simulink model "Copy_of_cantoni_combined_matrices_3pools_gates_hil"  (R2019b)
settings: Solver=FixedStepDiscrete  StartTime=0.0  StopTime=60*30  FixedStep=1/SPS  RelTol=1e-3
undefined symbols (not defined in the file or in its folder): ddelay, LF, Pd, Pd0, serial, SPS, Wis
libraries: instrumentlib x12, hdlsllib x4, simulink x4, sldrtlib x1
settings Model: Creator=Jacob  LastModifiedBy=bas
settings DataIOCC: ReturnWorkspaceOutputs=off
settings SFSimCC: CustomCodeUndefinedFunction=UseInterfaceOnly

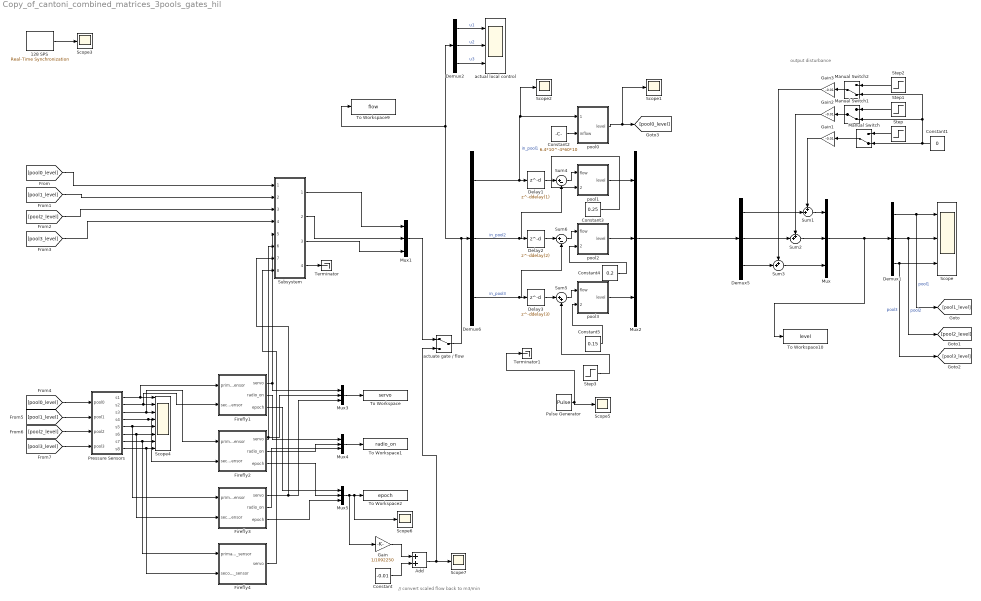
== system Copy_of_cantoni_combined_matrices_3pools_gates_hil ==
  note: // convert scaled flow back to m3/min
  note: output disturbance
  128 SPS : sldrtlib/Real-Time Synchronization  SampleTime=1/SPS  MaxMissedTicks=inf  ShowMissedTicks=on  YieldWhenWaiting=off
  Add : Sum
  Constant : Constant  Value=-0.01
  Constant1 : Constant  Value=0
  Constant2 : Constant  Value=6.4*10^-4*60*10
  Constant3 : Constant  Value=0.25  SampleTime=-1
  Constant4 : Constant  Value=0.2
  Constant5 : Constant  Value=0.15
  Delay1 : Delay  DelayLength=ddelay(1)
  Delay2 : Delay  DelayLength=ddelay(2)
  Delay3 : Delay  DelayLength=ddelay(3)
  Demux{1..2,5..6} (4 alike) : Demux  Outputs=3
  Firefly1 : Subsystem
  Firefly2 : Subsystem
  Firefly3 : Subsystem
  Firefly4 : Subsystem
  Gain : Gain  Gain=1/1092250
  Gain1 : Gain  Gain=-0.01
  Gain2 : Gain  Gain=-0.01
  Gain3 : Gain  Gain=-0.01
  Manual Switch : ManualSwitch  CurrentSetting=0
  Manual Switch1 : ManualSwitch  CurrentSetting=0
  Manual Switch2 : ManualSwitch  CurrentSetting=0
  Mux{,1..5} (6 alike) : Mux  Inputs=3
  Pressure Sensors : Subsystem
  Pulse Generator : DiscretePulseGenerator  Amplitude=-0.015  Period=60  PulseWidth=10
  Scope : Scope  NumInputPorts=3
  Scope{1..3,5..7} (6 alike) : Scope
  Scope4 : Scope  NumInputPorts=8
  Step : Step  Time=50  SampleTime=0
  Step1 : Step  Time=50  SampleTime=0
  Step2 : Step  Time=50  SampleTime=0
  Step3 : Step  Time=20  After=-0.015  SampleTime=0
  Subsystem : Subsystem
  Sum1 : Sum  Inputs=++|
  Sum2 : Sum  Inputs=++|
  Sum3 : Sum  Inputs=++|
  Sum4 : Sum  Inputs=|+-
  Sum5 : Sum  Inputs=|++
  Sum6 : Sum  Inputs=|+-
  Terminator : Terminator
  Terminator1 : Terminator
  To Workspace : ToWorkspace  VariableName=servo  SaveFormat=Timeseries  SampleTime=-1
  To Workspace1 : ToWorkspace  VariableName=radio_on  SaveFormat=Timeseries  SampleTime=-1
  To Workspace10 : ToWorkspace  VariableName=level  SaveFormat=Timeseries  SampleTime=-1
  To Workspace2 : ToWorkspace  VariableName=epoch  SaveFormat=Timeseries  SampleTime=-1
  To Workspace9 : ToWorkspace  VariableName=flow  SaveFormat=Timeseries  SampleTime=-1
  actual local control : Scope  NumInputPorts=3
  actuate gate / flow : ManualSwitch
  pool0 : Subsystem
  pool1 : Subsystem
  pool2 : Subsystem
  pool3 : Subsystem
  wires:
  Demux1/1 -> Scope/1, [pool1_level]  "pool1"
  Demux1/2 -> [pool2_level], Scope/2  "pool2"
  Demux1/3 -> [pool3_level], Scope/3  "pool3"
  Step/1 -> Manual Switch/1
  Sum1/1 -> Mux/1
  Sum2/1 -> Mux/2
  Gain2/1 -> Sum2/1
  Step1/1 -> Manual Switch1/1
  Gain1/1 -> Sum1/1
  Manual Switch/1 -> Gain1/1
  Constant1/1 -> Manual Switch1/2, Manual Switch2/2, Manual Switch/2
  Manual Switch1/1 -> Gain2/1
  Sum3/1 -> Mux/3
  Manual Switch2/1 -> Gain3/1
  Step2/1 -> Manual Switch2/1
  Gain3/1 -> Sum3/1
  Demux5/1 -> Sum1/2
  Demux5/2 -> Sum2/2
  Demux5/3 -> Sum3/2
  Delay1/1 -> Sum4/1
  Delay2/1 -> Sum6/1
  Demux6/1 -> Scope2/1, pool0/1(outflow), Delay1/1  "in_pool1"
  Demux6/2 -> Sum4/2, Delay2/1  "in_pool2"
  Demux6/3 -> Sum6/2, Delay3/1  "in_pool3"
  Sum4/1 -> pool1/1(flow)
  pool1/1(level) -> Mux2/1
  Sum6/1 -> pool2/1(flow)
  pool2/1(level) -> Mux2/2
  Delay3/1 -> Sum5/1
  pool3/1(level) -> Mux2/3
  Demux2/3 -> actual local control/3  "u3"
  Demux2/1 -> actual local control/1  "u1"
  Demux2/2 -> actual local control/2  "u2"
  actuate gate / flow/1 -> To Workspace9/1, Demux2/1, Demux6/1
  pool0/1(level) -> Scope1/1, [pool0_level]
  [pool0_level] -> Subsystem/1(pool0)
  [pool1_level] -> Subsystem/2(pool1)
  [pool2_level] -> Subsystem/3(pool2)
  [pool3_level] -> Subsystem/4(pool3)
  Constant2/1 -> pool0/2(inflow)
  Sum5/1 -> pool3/1(flow)
  Pulse Generator/1 -> Terminator1/1, Scope5/1
  Mux/1 -> To Workspace10/1, Demux1/1
  Pressure Sensors/1(s1) -> Firefly1/1(primary_sensor), Scope4/1
  Pressure Sensors/2(s2) -> Firefly1/2(secondary_sensor), Scope4/2
  Pressure Sensors/3(s3) -> Firefly2/1(primary_sensor), Scope4/3
  Pressure Sensors/4(s4) -> Firefly2/2(secondary_sensor), Scope4/4
  Pressure Sensors/5(s5) -> Firefly3/1(primary_sensor), Scope4/5
  Pressure Sensors/6(s6) -> Firefly3/2(secondary_sensor), Scope4/6
  Pressure Sensors/7(s7) -> Firefly4/1(primary_sensor), Scope4/7
  Pressure Sensors/8(s8) -> Firefly4/2(secondary_sensor), Scope4/8
  [pool0_level] -> Pressure Sensors/1(pool0)
  [pool1_level] -> Pressure Sensors/2(pool1)
  [pool2_level] -> Pressure Sensors/3(pool2)
  [pool3_level] -> Pressure Sensors/4(pool3)
  Subsystem/1(flow0_1) -> Mux1/1
  Subsystem/2(flow1_2) -> Mux1/2
  Subsystem/3(flow2_3) -> Mux1/3
  Subsystem/4(flow3_4) -> Terminator/1
  Mux2/1 -> Demux5/1
  Firefly1/1("servo ") -> Subsystem/5(servo1), Mux3/1
  Firefly4/1("servo ") -> Subsystem/8(servo4)
  128 SPS/1 -> Scope3/1
  Constant5/1 -> pool3/2("initail_level ")
  Constant4/1 -> pool2/2(initial_level)
  Constant3/1 -> pool1/2(initial_level)
  Firefly3/1("servo ") -> Mux3/3, Subsystem/7(servo3)
  Mux3/1 -> To Workspace/1
  Mux4/1 -> To Workspace1/1
  Mux5/1 -> Gain/1, Scope6/1, To Workspace2/1
  Firefly1/2(radio_on) -> Mux4/1
  Firefly1/3(epoch) -> Mux5/1
  Firefly2/1("servo ") -> Mux3/2, Subsystem/6(servo2)
  Firefly2/2(radio_on) -> Mux4/2
  Firefly2/3(epoch) -> Mux5/2
  Firefly3/2(radio_on) -> Mux4/3
  Firefly3/3(epoch) -> Mux5/3
  Step3/1 -> Sum5/2
  Gain/1 -> Add/1
  Constant/1 -> Add/2
  Add/1 -> actuate gate / flow/2, Scope7/1
  Mux1/1 -> actuate gate / flow/1

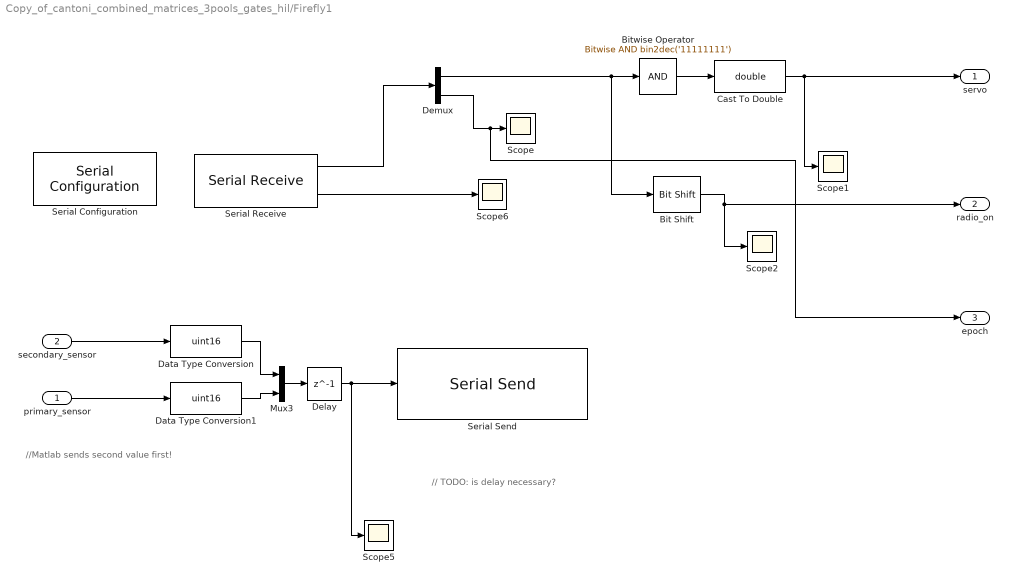
== system Copy_of_cantoni_combined_matrices_3pools_gates_hil/Firefly1 ==
  note: // TODO: is delay necessary?
  note: //Matlab sends second value first!
  primary_sensor : Inport
  secondary_sensor : Inport  Port=2
  Bit Shift : hdlsllib/Logic and Bit Operations/Bit Shift  mode=Shift Right Logical  N=8
      settings: SourceProductName=Simulink
  Bitwise Operator : simulink/Logic and Bit Operations/Bitwise Operator  logicop=AND  UseBitMask=on  BitMask=bin2dec('11111111')  BitMaskRealWorld=Stored Integer
  Cast To Double : DataTypeConversion  OutDataTypeStr=double
  Data Type Conversion : DataTypeConversion  OutDataTypeStr=uint16
  Data Type Conversion1 : DataTypeConversion  OutDataTypeStr=uint16
  Delay : Delay  DelayLength=1
  Demux : Demux  Outputs=2
  Mux3 : Mux  Inputs=2
  Scope{,1..2,5..6} (5 alike) : Scope
  Serial Configuration : instrumentlib/Serial Configuration  Priority=-200000  ComPortMenu=<Please select a port...>  ComPort=/dev/cu.SLAB_USBtoUART  ObjConstructor=serial('/dev/cu.SLAB_USBtoUART');  BaudRate=460800  DataBits=8  Parity=none  StopBits=1  FlowControl=none  Timeout=10  ByteOrder=BigEndian
  Serial Receive : instrumentlib/Serial Receive  ComPortMenu=<Please select a port...>  ComPort=/dev/cu.SLAB_USBtoUART  ObjConstructor=serial('/dev/cu.SLAB_USBtoUART');  Terminator=<none>  DataSize="[2  1]"  DataType=uint16  EnableBlockingMode=off  ActionDataUnavailable=Output last received value  CustomValue=0  SampleTime=1/SPS
  Serial Send : instrumentlib/Serial Send  ComPortMenu=<Please select a port...>  ComPort=/dev/cu.SLAB_USBtoUART  ObjConstructor=serial('/dev/cu.SLAB_USBtoUART');  Header=#  Terminator=LF ('\n')  EnableBlockingMode=off
  "servo " : Outport
  radio_on : Outport  Port=2
  epoch : Outport  Port=3
  wires:
  Data Type Conversion1/1 -> Mux3/2
  primary_sensor/1 -> Data Type Conversion1/1
  secondary_sensor/1 -> Data Type Conversion/1
  Serial Receive/2 -> Scope6/1
  Mux3/1 -> Delay/1
  Delay/1 -> Serial Send/1, Scope5/1
  Data Type Conversion/1 -> Mux3/1
  Demux/2 -> epoch/1, Scope/1
  Serial Receive/1 -> Demux/1
  Cast To Double/1 -> Scope1/1, "servo "/1
  Demux/1 -> Bit Shift/1, Bitwise Operator/1
  Bitwise Operator/1 -> Cast To Double/1
  Bit Shift/1 -> radio_on/1, Scope2/1

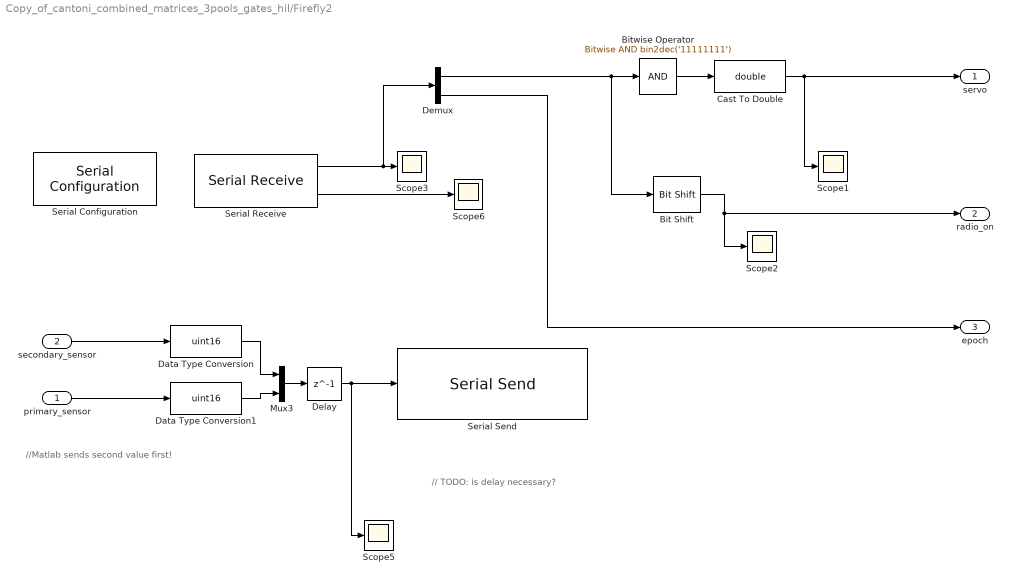
== system Copy_of_cantoni_combined_matrices_3pools_gates_hil/Firefly2 ==
  note: // TODO: is delay necessary?
  note: //Matlab sends second value first!
  primary_sensor : Inport
  secondary_sensor : Inport  Port=2
  Bit Shift : hdlsllib/Logic and Bit Operations/Bit Shift  mode=Shift Right Logical  N=8
      settings: SourceProductName=Simulink
  Bitwise Operator : simulink/Logic and Bit Operations/Bitwise Operator  logicop=AND  UseBitMask=on  BitMask=bin2dec('11111111')  BitMaskRealWorld=Stored Integer
  Cast To Double : DataTypeConversion  OutDataTypeStr=double
  Data Type Conversion : DataTypeConversion  OutDataTypeStr=uint16
  Data Type Conversion1 : DataTypeConversion  OutDataTypeStr=uint16
  Delay : Delay  DelayLength=1
  Demux : Demux  Outputs=2
  Mux3 : Mux  Inputs=2
  Scope{1..3,5..6} (5 alike) : Scope
  Serial Configuration : instrumentlib/Serial Configuration  Priority=-200000  ComPortMenu=<Please select a port...>  ComPort=/dev/cu.SLAB_USBtoUART4  ObjConstructor=serial('/dev/cu.SLAB_USBtoUART4');  BaudRate=460800  DataBits=8  Parity=none  StopBits=1  FlowControl=none  Timeout=10  ByteOrder=BigEndian
  Serial Receive : instrumentlib/Serial Receive  ComPortMenu=<Please select a port...>  ComPort=/dev/cu.SLAB_USBtoUART4  ObjConstructor=serial('/dev/cu.SLAB_USBtoUART4');  Terminator=<none>  DataSize="[2  1]"  DataType=uint16  EnableBlockingMode=off  ActionDataUnavailable=Output last received value  CustomValue=0  SampleTime=1/SPS
  Serial Send : instrumentlib/Serial Send  ComPortMenu=<Please select a port...>  ComPort=/dev/cu.SLAB_USBtoUART4  ObjConstructor=serial('/dev/cu.SLAB_USBtoUART4');  Header=#  Terminator=LF ('\n')  EnableBlockingMode=off
  "servo " : Outport
  radio_on : Outport  Port=2
  epoch : Outport  Port=3
  wires:
  Data Type Conversion1/1 -> Mux3/2
  primary_sensor/1 -> Data Type Conversion1/1
  secondary_sensor/1 -> Data Type Conversion/1
  Serial Receive/2 -> Scope6/1
  Mux3/1 -> Delay/1
  Delay/1 -> Serial Send/1, Scope5/1
  Data Type Conversion/1 -> Mux3/1
  Serial Receive/1 -> Demux/1, Scope3/1
  Cast To Double/1 -> Scope1/1, "servo "/1
  Demux/1 -> Bit Shift/1, Bitwise Operator/1
  Bitwise Operator/1 -> Cast To Double/1
  Demux/2 -> epoch/1
  Bit Shift/1 -> radio_on/1, Scope2/1

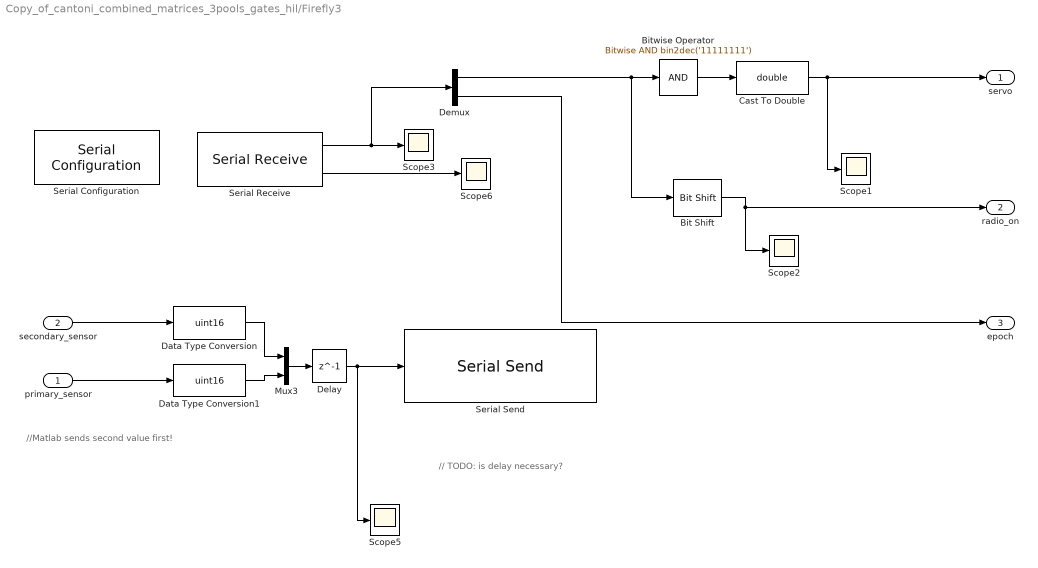
== system Copy_of_cantoni_combined_matrices_3pools_gates_hil/Firefly3 ==
  note: // TODO: is delay necessary?
  note: //Matlab sends second value first!
  primary_sensor : Inport
  secondary_sensor : Inport  Port=2
  Bit Shift : hdlsllib/Logic and Bit Operations/Bit Shift  mode=Shift Right Logical  N=8
      settings: SourceProductName=Simulink
  Bitwise Operator : simulink/Logic and Bit Operations/Bitwise Operator  logicop=AND  UseBitMask=on  BitMask=bin2dec('11111111')  BitMaskRealWorld=Stored Integer
  Cast To Double : DataTypeConversion  OutDataTypeStr=double
  Data Type Conversion : DataTypeConversion  OutDataTypeStr=uint16
  Data Type Conversion1 : DataTypeConversion  OutDataTypeStr=uint16
  Delay : Delay  DelayLength=1
  Demux : Demux  Outputs=2
  Mux3 : Mux  Inputs=2
  Scope{1..3,5..6} (5 alike) : Scope
  Serial Configuration : instrumentlib/Serial Configuration  Priority=-200000  ComPortMenu=<Please select a port...>  ComPort=/dev/cu.SLAB_USBtoUART6  ObjConstructor=serial('/dev/cu.SLAB_USBtoUART6');  BaudRate=460800  DataBits=8  Parity=none  StopBits=1  FlowControl=none  Timeout=10  ByteOrder=BigEndian
  Serial Receive : instrumentlib/Serial Receive  ComPortMenu=<Please select a port...>  ComPort=/dev/cu.SLAB_USBtoUART6  ObjConstructor=serial('/dev/cu.SLAB_USBtoUART6');  Terminator=<none>  DataSize="[2  1]"  DataType=uint16  EnableBlockingMode=off  ActionDataUnavailable=Output last received value  CustomValue=0  SampleTime=1/SPS
  Serial Send : instrumentlib/Serial Send  ComPortMenu=<Please select a port...>  ComPort=/dev/cu.SLAB_USBtoUART6  ObjConstructor=serial('/dev/cu.SLAB_USBtoUART6');  Header=#  Terminator=LF ('\n')  EnableBlockingMode=off
  "servo " : Outport
  radio_on : Outport  Port=2
  epoch : Outport  Port=3
  wires:
  Serial Receive/1 -> Demux/1, Scope3/1
  Data Type Conversion1/1 -> Mux3/2
  primary_sensor/1 -> Data Type Conversion1/1
  secondary_sensor/1 -> Data Type Conversion/1
  Serial Receive/2 -> Scope6/1
  Mux3/1 -> Delay/1
  Delay/1 -> Serial Send/1, Scope5/1
  Data Type Conversion/1 -> Mux3/1
  Cast To Double/1 -> Scope1/1, "servo "/1
  Demux/1 -> Bit Shift/1, Bitwise Operator/1
  Bitwise Operator/1 -> Cast To Double/1
  Demux/2 -> epoch/1
  Bit Shift/1 -> radio_on/1, Scope2/1

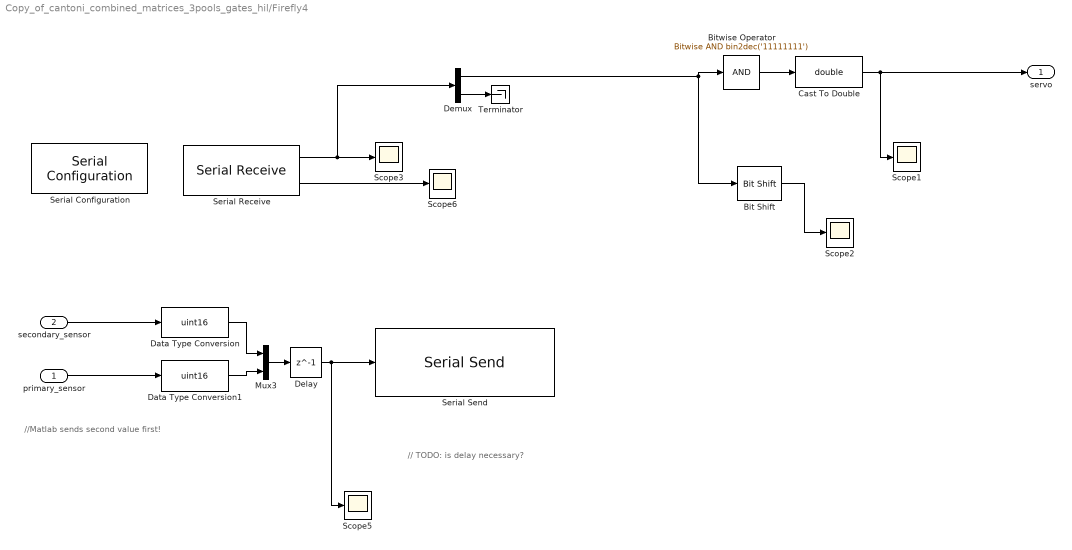
== system Copy_of_cantoni_combined_matrices_3pools_gates_hil/Firefly4 ==
  note: // TODO: is delay necessary?
  note: //Matlab sends second value first!
  primary_sensor : Inport
  secondary_sensor : Inport  Port=2
  Bit Shift : hdlsllib/Logic and Bit Operations/Bit Shift  mode=Shift Right Logical  N=8
      settings: SourceProductName=Simulink
  Bitwise Operator : simulink/Logic and Bit Operations/Bitwise Operator  logicop=AND  UseBitMask=on  BitMask=bin2dec('11111111')  BitMaskRealWorld=Stored Integer
  Cast To Double : DataTypeConversion  OutDataTypeStr=double
  Data Type Conversion : DataTypeConversion  OutDataTypeStr=uint16
  Data Type Conversion1 : DataTypeConversion  OutDataTypeStr=uint16
  Delay : Delay  DelayLength=1
  Demux : Demux  Outputs=2
  Mux3 : Mux  Inputs=2
  Scope{1..3,5..6} (5 alike) : Scope
  Serial Configuration : instrumentlib/Serial Configuration  Priority=-200000  ComPortMenu=<Please select a port...>  ComPort=/dev/cu.SLAB_USBtoUART8  ObjConstructor=serial('/dev/cu.SLAB_USBtoUART8');  BaudRate=460800  DataBits=8  Parity=none  StopBits=1  FlowControl=none  Timeout=10  ByteOrder=BigEndian
  Serial Receive : instrumentlib/Serial Receive  ComPortMenu=<Please select a port...>  ComPort=/dev/cu.SLAB_USBtoUART8  ObjConstructor=serial('/dev/cu.SLAB_USBtoUART8');  Terminator=<none>  DataSize="[2  1]"  DataType=uint16  EnableBlockingMode=off  ActionDataUnavailable=Output last received value  CustomValue=0  SampleTime=1/SPS
  Serial Send : instrumentlib/Serial Send  ComPortMenu=<Please select a port...>  ComPort=/dev/cu.SLAB_USBtoUART8  ObjConstructor=serial('/dev/cu.SLAB_USBtoUART8');  Header=#  Terminator=LF ('\n')  EnableBlockingMode=off
  Terminator : Terminator
  "servo " : Outport
  wires:
  Serial Receive/1 -> Demux/1, Scope3/1
  Data Type Conversion1/1 -> Mux3/2
  primary_sensor/1 -> Data Type Conversion1/1
  secondary_sensor/1 -> Data Type Conversion/1
  Serial Receive/2 -> Scope6/1
  Mux3/1 -> Delay/1
  Delay/1 -> Serial Send/1, Scope5/1
  Data Type Conversion/1 -> Mux3/1
  Demux/2 -> Terminator/1
  Cast To Double/1 -> Scope1/1, "servo "/1
  Demux/1 -> Bitwise Operator/1, Bit Shift/1
  Bit Shift/1 -> Scope2/1
  Bitwise Operator/1 -> Cast To Double/1

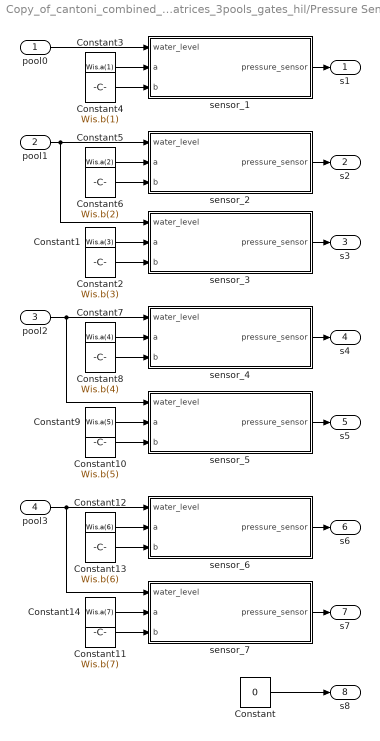
== system Copy_of_cantoni_combined_matrices_3pools_gates_hil/Pressure Sensors ==
  pool0 : Inport
  pool1 : Inport  Port=2
  pool2 : Inport  Port=3
  pool3 : Inport  Port=4
  Constant : Constant  Value=0
  Constant1 : Constant  Value=Wis.a(3)
  Constant10 : Constant  Value=Wis.b(5)
  Constant11 : Constant  Value=Wis.b(7)
  Constant12 : Constant  Value=Wis.a(6)
  Constant13 : Constant  Value=Wis.b(6)
  Constant14 : Constant  Value=Wis.a(7)
  Constant2 : Constant  Value=Wis.b(3)
  Constant3 : Constant  Value=Wis.a(1)
  Constant4 : Constant  Value=Wis.b(1)
  Constant5 : Constant  Value=Wis.a(2)
  Constant6 : Constant  Value=Wis.b(2)
  Constant7 : Constant  Value=Wis.a(4)
  Constant8 : Constant  Value=Wis.b(4)
  Constant9 : Constant  Value=Wis.a(5)
  sensor_1 : MATLAB Function  TreatAsAtomicUnit=on
  sensor_2 : MATLAB Function  TreatAsAtomicUnit=on
  sensor_3 : MATLAB Function  TreatAsAtomicUnit=on
  sensor_4 : MATLAB Function  TreatAsAtomicUnit=on
  sensor_5 : MATLAB Function  TreatAsAtomicUnit=on
  sensor_6 : MATLAB Function  TreatAsAtomicUnit=on
  sensor_7 : MATLAB Function  TreatAsAtomicUnit=on
  s1 : Outport
  s2 : Outport  Port=2
  s3 : Outport  Port=3
  s4 : Outport  Port=4
  s5 : Outport  Port=5
  s6 : Outport  Port=6
  s7 : Outport  Port=7
  s8 : Outport  Port=8
  wires:
  sensor_1/1(pressure_sensor) -> s1/1
  Constant5/1 -> sensor_2/2(a)
  Constant3/1 -> sensor_1/2(a)
  Constant4/1 -> sensor_1/3(b)
  Constant6/1 -> sensor_2/3(b)
  sensor_2/1(pressure_sensor) -> s2/1
  pool0/1 -> sensor_1/1(water_level)
  Constant1/1 -> sensor_3/2(a)
  Constant2/1 -> sensor_3/3(b)
  sensor_3/1(pressure_sensor) -> s3/1
  sensor_4/1(pressure_sensor) -> s4/1
  Constant7/1 -> sensor_4/2(a)
  Constant8/1 -> sensor_4/3(b)
  Constant10/1 -> sensor_5/3(b)
  Constant9/1 -> sensor_5/2(a)
  pool2/1 -> sensor_5/1(water_level), sensor_4/1(water_level)
  sensor_5/1(pressure_sensor) -> s5/1
  Constant12/1 -> sensor_6/2(a)
  pool3/1 -> sensor_7/1(water_level), sensor_6/1(water_level)
  sensor_6/1(pressure_sensor) -> s6/1
  Constant13/1 -> sensor_6/3(b)
  Constant11/1 -> sensor_7/3(b)
  Constant14/1 -> sensor_7/2(a)
  sensor_7/1(pressure_sensor) -> s7/1
  Constant/1 -> s8/1
  pool1/1 -> sensor_3/1(water_level), sensor_2/1(water_level)

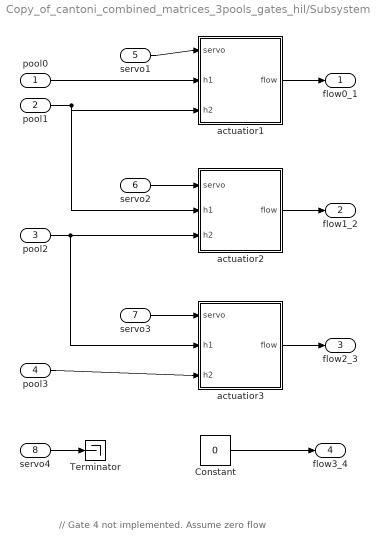
== system Copy_of_cantoni_combined_matrices_3pools_gates_hil/Subsystem ==
  note: // Gate 4 not implemented. Assume zero flow
  pool0 : Inport
  pool1 : Inport  Port=2
  pool2 : Inport  Port=3
  pool3 : Inport  Port=4
  servo1 : Inport  Port=5
  servo2 : Inport  Port=6
  servo3 : Inport  Port=7
  servo4 : Inport  Port=8
  Constant : Constant  Value=0
  Terminator : Terminator
  actuatior1 : MATLAB Function  TreatAsAtomicUnit=on
  actuatior2 : MATLAB Function  TreatAsAtomicUnit=on
  actuatior3 : MATLAB Function  TreatAsAtomicUnit=on
  flow0_1 : Outport
  flow1_2 : Outport  Port=2
  flow2_3 : Outport  Port=3
  flow3_4 : Outport  Port=4
  wires:
  pool1/1 -> actuatior2/2(h1), actuatior1/3(h2)
  servo2/1 -> actuatior2/1(servo)
  pool2/1 -> actuatior3/2(h1), actuatior2/3(h2)
  actuatior1/1(flow) -> flow0_1/1
  servo1/1 -> actuatior1/1(servo)
  servo3/1 -> actuatior3/1(servo)
  pool0/1 -> actuatior1/2(h1)
  actuatior2/1(flow) -> flow1_2/1
  pool3/1 -> actuatior3/3(h2)
  actuatior3/1(flow) -> flow2_3/1
  servo4/1 -> Terminator/1
  Constant/1 -> flow3_4/1

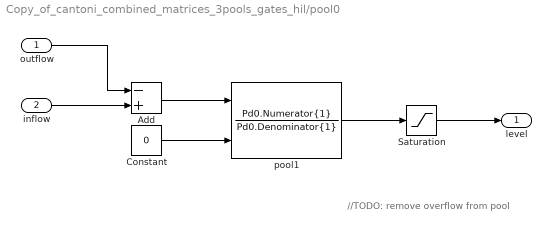
== system Copy_of_cantoni_combined_matrices_3pools_gates_hil/pool0 ==
  note: //TODO: remove overflow from pool
  outflow : Inport
  inflow : Inport  Port=2
  Add : Sum  Inputs=-+
  Constant : Constant  Value=0
  Saturation : Saturate  UpperLimit=0.3
  pool1 : DiscreteTransferFcn  Numerator=Pd0.Numerator{1}  Denominator=Pd0.Denominator{1}  InitialStatesSource=Input port
      settings: InputPortMap=u0,p5
  level : Outport
  wires:
  pool1/1 -> Saturation/1
  outflow/1 -> Add/1
  inflow/1 -> Add/2
  Add/1 -> pool1/1
  Constant/1 -> pool1/2
  Saturation/1 -> level/1

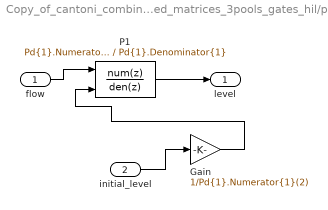
== system Copy_of_cantoni_combined_matrices_3pools_gates_hil/pool1 ==
  flow : Inport
  initial_level : Inport  Port=2
  Gain : Gain  Gain=1/Pd{1}.Numerator{1}(2)
  P1 : DiscreteTransferFcn  Numerator=Pd{1}.Numerator{1}  Denominator=Pd{1}.Denominator{1}  InitialStatesSource=Input port
      settings: InputPortMap=u0,p5
  level : Outport
  wires:
  flow/1 -> P1/1
  P1/1 -> level/1
  Gain/1 -> P1/2
  initial_level/1 -> Gain/1

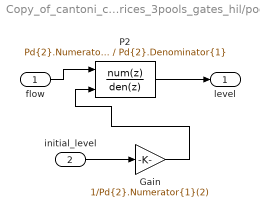
== system Copy_of_cantoni_combined_matrices_3pools_gates_hil/pool2 ==
  flow : Inport
  initial_level : Inport  Port=2
  Gain : Gain  Gain=1/Pd{2}.Numerator{1}(2)
  P2 : DiscreteTransferFcn  Numerator=Pd{2}.Numerator{1}  Denominator=Pd{2}.Denominator{1}  InitialStatesSource=Input port
      settings: InputPortMap=u0,p5
  level : Outport
  wires:
  flow/1 -> P2/1
  P2/1 -> level/1
  Gain/1 -> P2/2
  initial_level/1 -> Gain/1

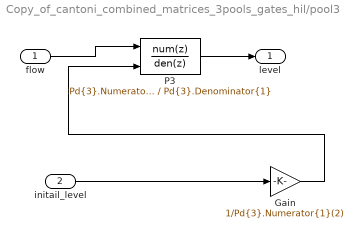
== system Copy_of_cantoni_combined_matrices_3pools_gates_hil/pool3 ==
  flow : Inport
  "initail_level " : Inport  Port=2
  Gain : Gain  Gain=1/Pd{3}.Numerator{1}(2)
  P3 : DiscreteTransferFcn  Numerator=Pd{3}.Numerator{1}  Denominator=Pd{3}.Denominator{1}  InitialStatesSource=Input port
      settings: InputPortMap=u0,p5
  level : Outport
  wires:
  P3/1 -> level/1
  flow/1 -> P3/1
  Gain/1 -> P3/2
  "initail_level "/1 -> Gain/1

== matlab function Copy_of_cantoni_combined_matrices_3pools_gates_hil/Pressure Sensors/sensor_1 ==
  data: water_level input; pressure_sensor output; a input; b input
function pressure_sensor = fcn(water_level, a, b)

pressure_sensor = m2pressure(water_level, a, b);

== matlab function Copy_of_cantoni_combined_matrices_3pools_gates_hil/Pressure Sensors/sensor_2 ==
  data: water_level input; pressure_sensor output; a input; b input
function pressure_sensor = fcn(water_level, a, b)

pressure_sensor = m2pressure(water_level, a, b);

== matlab function Copy_of_cantoni_combined_matrices_3pools_gates_hil/Pressure Sensors/sensor_3 ==
  data: water_level input; pressure_sensor output; a input; b input
function pressure_sensor = fcn(water_level, a, b)

pressure_sensor = m2pressure(water_level, a, b);

== matlab function Copy_of_cantoni_combined_matrices_3pools_gates_hil/Pressure Sensors/sensor_4 ==
  data: water_level input; pressure_sensor output; a input; b input
function pressure_sensor = fcn(water_level, a, b)

pressure_sensor = m2pressure(water_level, a, b);

== matlab function Copy_of_cantoni_combined_matrices_3pools_gates_hil/Pressure Sensors/sensor_5 ==
  data: water_level input; pressure_sensor output; a input; b input
function pressure_sensor = fcn(water_level, a, b)

pressure_sensor = m2pressure(water_level, a, b);

== matlab function Copy_of_cantoni_combined_matrices_3pools_gates_hil/Pressure Sensors/sensor_6 ==
  data: water_level input; pressure_sensor output; a input; b input
function pressure_sensor = fcn(water_level, a, b)

pressure_sensor = m2pressure(water_level, a, b);

== matlab function Copy_of_cantoni_combined_matrices_3pools_gates_hil/Pressure Sensors/sensor_7 ==
  data: water_level input; pressure_sensor output; a input; b input
function pressure_sensor = fcn(water_level, a, b)

pressure_sensor = m2pressure(water_level, a, b);

== matlab function Copy_of_cantoni_combined_matrices_3pools_gates_hil/Subsystem/actuatior1 ==
  data: servo input; flow output; h1 input; h2 input
function flow = fcn(servo, h1, h2)

flow = gate2flow(servo, h1, h2);

== matlab function Copy_of_cantoni_combined_matrices_3pools_gates_hil/Subsystem/actuatior2 ==
  data: servo input; flow output; h1 input; h2 input
function flow = fcn(servo, h1, h2)

flow = gate2flow(servo, h1, h2);

== matlab function Copy_of_cantoni_combined_matrices_3pools_gates_hil/Subsystem/actuatior3 ==
  data: servo input; flow output; h1 input; h2 input
function flow = fcn(servo, h1, h2)

flow = gate2flow(servo, h1, h2);
